simulink model "Both_Test_v3"  (R2017b)
settings: Solver=VariableStepAuto  StartTime=0.0  StopTime=2  MaxStep=1e-4  RelTol=1e-3
undefined symbols (not defined in the file): sigbuilder_block
libraries: powerlib x18, nesl_utility x2, fl_lib x2, simulink x1
settings Model: Creator=paul.rogers  LastModifiedBy=acer8_000
settings OptimizationCC: BlockReduction=off  ConditionallyExecuteInputs=off  DefaultParameterBehavior=Inlined
settings DebuggingCC: AlgebraicLoopMsg=error  SingleTaskRateTransMsg=error
settings HardwareCC: ProdBitPerPointer=32  ProdBitPerSizeT=32  ProdBitPerPtrDiffT=32  ProdLargestAtomicFloat=None  ProdIntDivRoundTo=Undefined  ProdEndianess=Unspecified  ProdWordSize=32  ProdHWDeviceType=ASIC/FPGA->ASIC/FPGA  ProdEqTarget=off
settings CodeAppCC: StateflowObjectComments=on
settings SimscapeCC: SimscapeNormalizeSystem=off

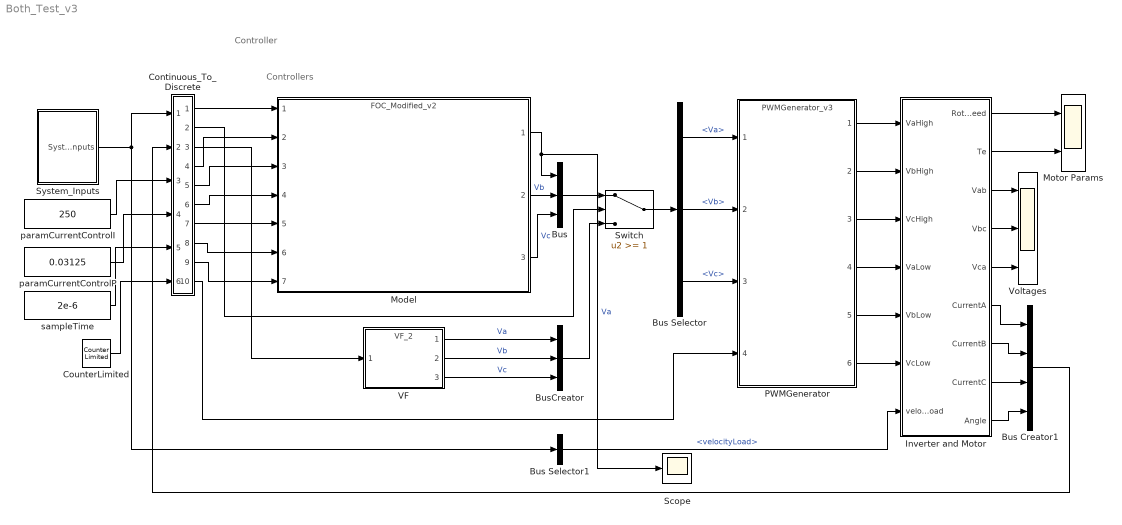
== system Both_Test_v3 ==
  note: Controllers
  note: Controller
  Bus : BusCreator  Inputs=3
  Bus Creator1 : BusCreator  Inputs=4
  Bus Selector : BusSelector  OutputSignals=Va,Vb,Vc
  Bus Selector1 : BusSelector  OutputSignals=velocityLoad
  BusCreator : BusCreator  Inputs=3
  Continuous_To_Discrete : Subsystem
      mask Display: fprintf('C/D')
  CounterLimited : simulink/Sources/Counter Limited  uplimit=50  tsamp=1e-5
  Inverter and Motor : Subsystem
  Model : ModelReference  ModelNameDialog=FOC_Modified_v2.slx  SimulationMode=Normal  ModelReferenceVersion=1.83
  Motor Params : Scope  NumInputPorts=2
  PWMGenerator : ModelReference  ModelNameDialog=PWMGenerator_v3.slx  SimulationMode=Normal  ModelReferenceVersion=1.20
  Scope : Scope
  Switch : Switch  Threshold=1
  System_Inputs : Subsystem  Description=""
      mask Display: disp('System\nInputs')
  VF : ModelReference  ModelNameDialog=VF_2.slx  SimulationMode=Normal  ModelReferenceVersion=1.58
  "Voltages " : Scope  NumInputPorts=3
  paramCurrentControlI : Constant  Value=250  OutDataTypeStr=fixdt(1,16,3)
  paramCurrentControlP : Constant  Value=0.03125  OutDataTypeStr=fixdt(1,16,8)
  sampleTime : Constant  Value=2e-6  OutDataTypeStr=fixdt(1,16,30)
  wires:
  Inverter and Motor/9(Angle) -> Bus Creator1/4
  Inverter and Motor/8(CurrentC) -> Bus Creator1/3
  Inverter and Motor/6(CurrentA) -> Bus Creator1/1
  Inverter and Motor/7(CurrentB) -> Bus Creator1/2
  paramCurrentControlP/1 -> Continuous_To_Discrete/4(paramCurrentControlP)
  paramCurrentControlI/1 -> Continuous_To_Discrete/3(paramCurrentControlI)
  System_Inputs/1(System_Inputs) -> Continuous_To_Discrete/1(System_Inputs), Bus Selector1/1
  Bus Creator1/1 -> Continuous_To_Discrete/2(Motor_Measurements)
  sampleTime/1 -> Continuous_To_Discrete/5(sampleTime)
  Bus Selector1/1 -> Inverter and Motor/7(velocityLoad)  "<velocityLoad>"
  Inverter and Motor/2(Te) -> Motor Params/2
  Inverter and Motor/1(Rotor Speed) -> Motor Params/1
  Inverter and Motor/3(Vab) -> "Voltages "/1
  Inverter and Motor/4(Vbc) -> "Voltages "/2
  Inverter and Motor/5(Vca) -> "Voltages "/3
  PWMGenerator/1 -> Inverter and Motor/1(VaHigh)
  PWMGenerator/2 -> Inverter and Motor/2(VbHigh)
  PWMGenerator/3 -> Inverter and Motor/3(VcHigh)
  PWMGenerator/4 -> Inverter and Motor/4(VaLow)
  PWMGenerator/5 -> Inverter and Motor/5(VbLow)
  PWMGenerator/6 -> Inverter and Motor/6(VcLow)
  CounterLimited/1 -> Continuous_To_Discrete/6(Counter)
  Continuous_To_Discrete/10(Counter_timed) -> PWMGenerator/4
  Switch/1 -> Bus Selector/1
  Bus Selector/3 -> PWMGenerator/3  "<Vc>"
  Bus Selector/1 -> PWMGenerator/1  "<Va>"
  Bus Selector/2 -> PWMGenerator/2  "<Vb>"
  Bus/1 -> Switch/1
  Model/1 -> Scope/1, Bus/1  "Va"
  Model/2 -> Bus/2  "Vb"
  Model/3 -> Bus/3  "Vc"
  Continuous_To_Discrete/9(sampleTime_timed) -> Model/7
  Continuous_To_Discrete/8(paramCurrentControlP_timed) -> Model/6
  Continuous_To_Discrete/7(paramCurrentControlI_timed) -> Model/5
  Continuous_To_Discrete/6(Electrical_Position) -> Model/4
  Continuous_To_Discrete/5(Phase_Current_B) -> Model/3
  Continuous_To_Discrete/4(Phase_Current_A) -> Model/2
  Continuous_To_Discrete/1(Current_Command) -> Model/1
  Continuous_To_Discrete/3(Frequency) -> VF/1
  Continuous_To_Discrete/2(Switch) -> Switch/2
  VF/3 -> BusCreator/3  "Vc"
  VF/2 -> BusCreator/2  "Vb"
  BusCreator/1 -> Switch/3
  VF/1 -> BusCreator/1  "Va"

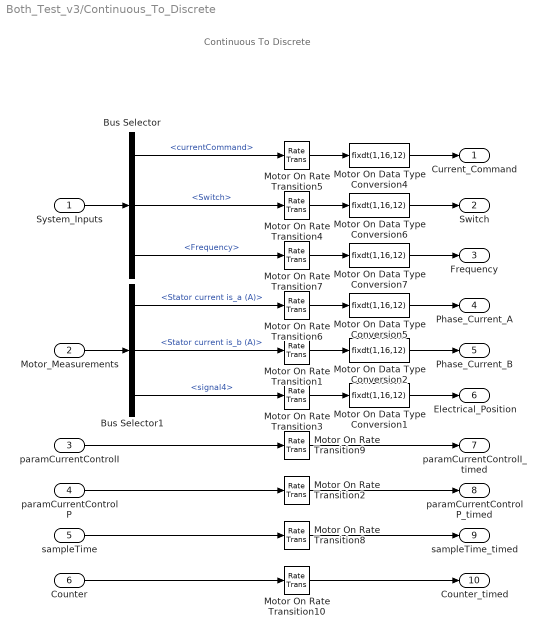
== system Both_Test_v3/Continuous_To_Discrete ==
  note: Continuous To Discrete
  System_Inputs : Inport
  Motor_Measurements : Inport  Port=2
  paramCurrentControlI : Inport  Port=3
  paramCurrentControlP : Inport  Port=4
  sampleTime : Inport  Port=5
  Counter : Inport  Port=6  OutDataTypeStr=uint8
  Bus Selector : BusSelector  OutputSignals=currentCommand,Switch,Frequency
  Bus Selector1 : BusSelector  OutputSignals=Stator current is_a (A),Stator current is_b (A),signal4
  Motor On Data Type Conversion{1..2,4..7} (6 alike) : DataTypeConversion  OutDataTypeStr=fixdt(1,16,12)
  Motor On Rate Transition{1..10} (10 alike) : RateTransition  Integrity=off  Deterministic=off  OutPortSampleTime=2e-6
  Current_Command : Outport
  Switch : Outport  Port=2
  Frequency : Outport  Port=3
  Phase_Current_A : Outport  Port=4
  Phase_Current_B : Outport  Port=5
  Electrical_Position : Outport  Port=6
  paramCurrentControlI_timed : Outport  Port=7
  paramCurrentControlP_timed : Outport  Port=8
  sampleTime_timed : Outport  Port=9
  Counter_timed : Outport  Port=10
  wires:
  Bus Selector1/3 -> Motor On Rate Transition3/1  "<signal4>"
  Bus Selector1/2 -> Motor On Rate Transition1/1  "<Stator current is_b (A)>"
  Bus Selector1/1 -> Motor On Rate Transition6/1  "<Stator current is_a (A)>"
  Motor On Data Type Conversion4/1 -> Current_Command/1
  Motor On Rate Transition6/1 -> Motor On Data Type Conversion5/1
  Motor On Rate Transition5/1 -> Motor On Data Type Conversion4/1
  Bus Selector/1 -> Motor On Rate Transition5/1  "<currentCommand>"
  Motor On Rate Transition3/1 -> Motor On Data Type Conversion1/1
  System_Inputs/1 -> Bus Selector/1
  Motor_Measurements/1 -> Bus Selector1/1
  Motor On Rate Transition1/1 -> Motor On Data Type Conversion2/1
  Motor On Rate Transition4/1 -> Motor On Data Type Conversion6/1
  Bus Selector/2 -> Motor On Rate Transition4/1  "<Switch>"
  Motor On Rate Transition7/1 -> Motor On Data Type Conversion7/1
  Bus Selector/3 -> Motor On Rate Transition7/1  "<Frequency>"
  Motor On Data Type Conversion6/1 -> Switch/1
  Motor On Data Type Conversion7/1 -> Frequency/1
  Motor On Data Type Conversion1/1 -> Electrical_Position/1
  Motor On Data Type Conversion2/1 -> Phase_Current_B/1
  Motor On Data Type Conversion5/1 -> Phase_Current_A/1
  paramCurrentControlI/1 -> Motor On Rate Transition9/1
  paramCurrentControlP/1 -> Motor On Rate Transition2/1
  sampleTime/1 -> Motor On Rate Transition8/1
  Counter/1 -> Motor On Rate Transition10/1
  Motor On Rate Transition10/1 -> Counter_timed/1
  Motor On Rate Transition8/1 -> sampleTime_timed/1
  Motor On Rate Transition2/1 -> paramCurrentControlP_timed/1
  Motor On Rate Transition9/1 -> paramCurrentControlI_timed/1

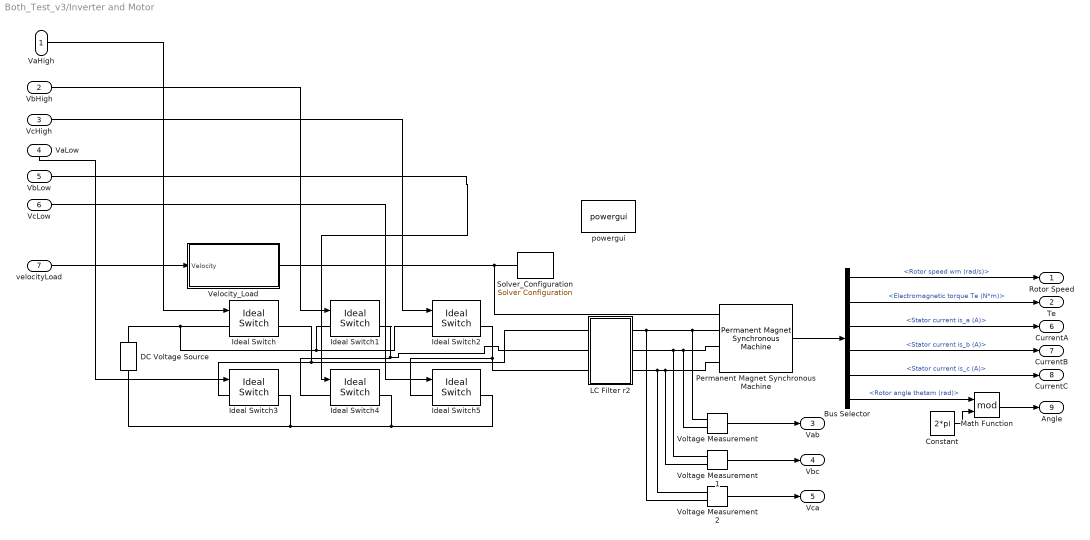
== system Both_Test_v3/Inverter and Motor ==
  VaHigh : Inport
  VbHigh : Inport  Port=2
  VcHigh : Inport  Port=3
  VaLow : Inport  Port=4
  VbLow : Inport  Port=5
  VcLow : Inport  Port=6
  velocityLoad : Inport  Port=7
  Bus Selector : BusSelector  OutputSignals=Rotor speed wm (rad/s),Electromagnetic torque Te (N*m),Stator current is_a (A),Stator current is_b (A),Stator current is_c (A),Rotor angle thetam (rad)
  Constant : Constant  Value=2*pi
  DC Voltage Source : powerlib/Electrical Sources/DC Voltage Source  Amplitude=42  Measurements=None
  Ideal Switch{,1..5} (6 alike) : powerlib/Power Electronics/Ideal Switch  Ron=0.001  Lon=0  IC=0  Rs=1e5  Cs=inf  Measurements=on
  LC Filter r2 : Subsystem  mask{L=10e-3, C=20e-6}
      mask prompts: L "Inductance"; C "Capacitance"
  Math Function : Math  Operator=mod  SaturateOnIntegerOverflow=on
  Permanent Magnet Synchronous Machine : powerlib/Machines/Permanent Magnet Synchronous Machine  NbPhases=3  FluxDistribution=Sinusoidal  RotorType=Salient-pole  MechanicalLoad=Mechanical rotational port  PresetModel=No  ShowDetailedParameters=on  MeasurementBus=off  Resistance=0.900000000000000  Inductance=8.5e-3  dqInductances=[0.001050000000000 0.001050000000000]  La=0.00049  MachineConstant=Torque Constant (N.m / A_peak)  Flux=0.005661  VoltageCst=4.1072  TorqueCst=0.033966007400000  Flat=120  Mechanical=[2.400927680000000e-06, 1.333630000000000e-05, 4, 0.002130661000000]  PolePairs=4  InitialConditions=[0,0, 0,0]  InitialConditions5ph=[0 0 0 0 0 0]  TsPowergui=0  TsBlock=-1  RefAngle=Aligned with phase A axis (original Park)
      settings: SourceProductName=Simscape Power Systems
  Solver_Configuration : nesl_utility/Solver Configuration  PhysicalDomain=network_engine_domain  SubClassName=solver  LeftPortType=input  RightPortType=generic  Accelerate=off  Tones=[]  Harmonics=[]  SimulateNoise=off  Profile=off  UseLocalSampling=off  EnableSwitchedLinearOptims=on  FrequencyDomain=off  UseCCode=off  RelTol=0.001  AbsTol=1e-06  MinStep=1e-09  ToWorkspace=off  RevertToSquareIcSolve=off  NumHomotopyIterations=100  PhasorMode=off  PhasorModeNumHarmonics=1  DoDC=off  ResidualTolerance=1e-9  UseLocalSolver=off  LocalSolverChoice=NE_BACKWARD_EULER_ADVANCER  LocalSolverSampleTime=.001  DoFixedCost=off  MaxNonlinIter=3  MaxModeIter=2  LinearAlgebra=Sparse  DelaysMemoryBudget=1024  AutomaticFiltering=on  FilteringTimeConstant=0.001
  Velocity_Load : Subsystem  VariantControl=loadType == motorLoad.disc
      mask Display:
      | image('hdlcoderVelocityLoadMask.png')
      | text(0.03, 0.5, '\omega', 'HorizontalAlignment', 'Left', 'texmode','on')
      | text(0.98, 0.5, 'R', 'HorizontalAlignment', 'Right')
  Voltage Measurement : powerlib/Measurements/Voltage Measurement  PhasorSimulation=off  OutputType=Complex  PSBequivalent=0
  Voltage Measurement1 : powerlib/Measurements/Voltage Measurement  PhasorSimulation=off  OutputType=Complex  PSBequivalent=0
  Voltage Measurement2 : powerlib/Measurements/Voltage Measurement  PhasorSimulation=off  OutputType=Complex  PSBequivalent=0
  powergui : powerlib/powergui  Priority=1  SimulationMode=Continuous  SampleTime=50e-6  frequency=60  Iterations=50  frequencyindice=0  Pbase=100e6  ErrMax=1e-4  UnitsV=kV  UnitsW=MW  buscounter=0  FunctionMessages=off  echomessages=off  EnableUseOfTLC=off  CurrentSourceSwitches=off  DisableSnubberDevices=off  DisableRonSwitches=off  DisableVfSwitches=off  DisplayEquations=off  SolverType=Tustin/Backward Euler (TBE)  Interpol=off  ExternalGateDelay=off  methode=off  Ts=100  x0status=blocks  SPID=on  SwTol=0  HookPort=off  RestoreLinks=warning  ResistiveCurrentMeasurement=off  Frange=[0:2:500]  Ylog=off  Xlog=on  ShowGrid=off  save=off  variable=ZData  structure=0  ZoomFFT=off  StartTime=0.0  cycles=1  DisplayStyle=1  fundamental=60  FreqAxis=off  MaxFrequency=1000  frequencyindicesteady=1  RmsSteady=1  display=off
  Rotor Speed : Outport
  Te : Outport  Port=2
  Vab : Outport  Port=3
  Vbc : Outport  Port=4
  Vca : Outport  Port=5
  CurrentA : Outport  Port=6
  CurrentB : Outport  Port=7
  CurrentC : Outport  Port=8
  Angle : Outport  Port=9
  wires:
  VbHigh/1 -> Ideal Switch1/1
  VcHigh/1 -> Ideal Switch2/1
  VcLow/1 -> Ideal Switch5/1
  VbLow/1 -> Ideal Switch4/1
  Permanent Magnet Synchronous Machine/1 -> Bus Selector/1
  Bus Selector/1 -> Rotor Speed/1  "<Rotor speed wm (rad/s)>"
  Bus Selector/2 -> Te/1  "<Electromagnetic torque Te (N*m)>"
  VaHigh/1 -> Ideal Switch/1
  Voltage Measurement2/1 -> Vca/1
  Voltage Measurement/1 -> Vab/1
  Voltage Measurement1/1 -> Vbc/1
  VaLow/1 -> Ideal Switch3/1
  Bus Selector/3 -> CurrentA/1  "<Stator current is_a (A)>"
  Bus Selector/4 -> CurrentB/1  "<Stator current is_b (A)>"
  Bus Selector/5 -> CurrentC/1  "<Stator current is_c (A)>"
  Bus Selector/6 -> Math Function/1  "<Rotor angle thetam (rad)>"
  Math Function/1 -> Angle/1
  Constant/1 -> Math Function/2
  velocityLoad/1 -> Velocity_Load/1(Velocity)
  connections:
  DC Voltage Source/RConn1 -- Ideal Switch2/LConn1 -- Ideal Switch1/LConn1 -- Ideal Switch/LConn1
  Ideal Switch2/RConn1 -- LC Filter r2/LConn3 -- Ideal Switch5/LConn1
  Ideal Switch1/RConn1 -- LC Filter r2/LConn2 -- Ideal Switch4/LConn1
  Ideal Switch/RConn1 -- LC Filter r2/LConn1 -- Ideal Switch3/LConn1
  DC Voltage Source/LConn1 -- Ideal Switch5/RConn1 -- Ideal Switch4/RConn1 -- Ideal Switch3/RConn1
  Solver_Configuration/RConn1 -- Permanent Magnet Synchronous Machine/LConn1 -- Velocity_Load/RConn1
  LC Filter r2/RConn1 -- Voltage Measurement2/LConn2 -- Voltage Measurement/LConn1 -- Permanent Magnet Synchronous Machine/LConn2
  LC Filter r2/RConn2 -- Voltage Measurement1/LConn1 -- Voltage Measurement/LConn2 -- Permanent Magnet Synchronous Machine/LConn3
  LC Filter r2/RConn3 -- Voltage Measurement2/LConn1 -- Voltage Measurement1/LConn2 -- Permanent Magnet Synchronous Machine/LConn4

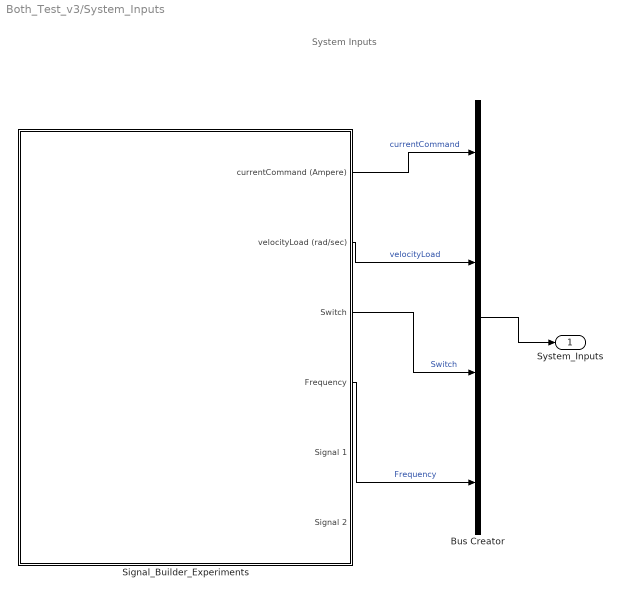
== system Both_Test_v3/System_Inputs ==
  note: System Inputs
  Bus Creator : BusCreator  Inputs=4
  Signal_Builder_Experiments : Subsystem  Tag=STV Subsys  LoadFcn=sigbuilder_block('load',[6 23.25 1428 723 ]);  StartFcn=sigbuilder_block('start');  StopFcn=sigbuilder_block('stop');  ClipboardFcn=sigbuilder_block('clipboard');  mask(Sigbuilder block){tuvar=[0:10]}
      mask init:
      | if ~strcmp(get_param(bdroot(gcb),'SimulationStatus'),'stopped'),tuvar = sigbuilder_block('maskInit'); end
      settings: CopyFcn=sigbuilder_block('copy');  DeleteFcn=sigbuilder_block('delete');  ModelCloseFcn=sigbuilder_block('modelClose');  PreSaveFcn=sigbuilder_block('preSave');  PauseFcn=sigbuilder_block('pause');  ContinueFcn=sigbuilder_block('continue');  NameChangeFcn=sigbuilder_block('namechange');  OpenFcn=sigbuilder_block('open',[6 23.25 1428 723 ]);  CloseFcn=sigbuilder_block('close');
      mask Display: plot(0, 0, 100, 100,[2, 2, 32, 32, 2], [68, 8, 8, 68, 68],[32, 2], [38, 38], [32, 19, 2],[53, 60, 44], [32, 17, 17, 2],[16, 16, 31, 31]);txt = getActiveGroup(gcbh);text(2, 100, txt,'verticalAlignment', 'top');
  System_Inputs : Outport
  wires:
  Signal_Builder_Experiments/2(velocityLoad (rad/sec)) -> Bus Creator/2  "velocityLoad"
  Signal_Builder_Experiments/1(currentCommand (Ampere)) -> Bus Creator/1  "currentCommand"
  Bus Creator/1 -> System_Inputs/1
  Signal_Builder_Experiments/3(Switch) -> Bus Creator/3  "Switch"
  Signal_Builder_Experiments/4(Frequency) -> Bus Creator/4  "Frequency"

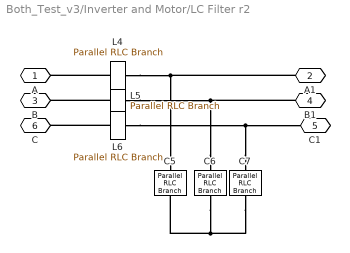
== system Both_Test_v3/Inverter and Motor/LC Filter r2 ==
  C5 : powerlib/Elements/Parallel RLC Branch  LConnTagsString=a  RConnTagsString=__new0  BranchType=C  Resistance=inf  Inductance=inf  SetiL0=off  InitialCurrent=0  Capacitance=C  Setx0=off  InitialVoltage=0  Measurements=None
  C6 : powerlib/Elements/Parallel RLC Branch  LConnTagsString=a  RConnTagsString=__new0  BranchType=C  Resistance=inf  Inductance=inf  SetiL0=off  InitialCurrent=0  Capacitance=C  Setx0=off  InitialVoltage=0  Measurements=None
  C7 : powerlib/Elements/Parallel RLC Branch  LConnTagsString=a  RConnTagsString=__new0  BranchType=C  Resistance=inf  Inductance=inf  SetiL0=off  InitialCurrent=0  Capacitance=C  Setx0=off  InitialVoltage=0  Measurements=None
  L4 : powerlib/Elements/Parallel RLC Branch  LConnTagsString=a  RConnTagsString=__new0  BranchType=L  Resistance=inf  Inductance=L  SetiL0=off  InitialCurrent=0  Capacitance=1.3e-3  Setx0=off  InitialVoltage=0  Measurements=None
  L5 : powerlib/Elements/Parallel RLC Branch  LConnTagsString=a  RConnTagsString=__new0  BranchType=L  Resistance=inf  Inductance=L  SetiL0=off  InitialCurrent=0  Capacitance=1.3e-3  Setx0=off  InitialVoltage=0  Measurements=None
  L6 : powerlib/Elements/Parallel RLC Branch  LConnTagsString=a  RConnTagsString=__new0  BranchType=L  Resistance=inf  Inductance=L  SetiL0=off  InitialCurrent=0  Capacitance=1.3e-3  Setx0=off  InitialVoltage=0  Measurements=None
  A : PMIOPort  Port=1  Side=Left
  A1 : PMIOPort  Port=2  Side=Right
  B : PMIOPort  Port=3  Side=Left
  B1 : PMIOPort  Port=4  Side=Right
  C1 : PMIOPort  Port=5  Side=Right
  C : PMIOPort  Port=6  Side=Left
  connections:
  L4/LConn1 -- A/RConn1
  L6/LConn1 -- C/RConn1
  C5/RConn1 -- C7/RConn1 -- C6/RConn1
  L5/LConn1 -- B/RConn1
  C6/LConn1 -- B1/RConn1 -- L5/RConn1
  L4/RConn1 -- A1/RConn1 -- C5/LConn1
  C7/LConn1 -- C1/RConn1 -- L6/RConn1

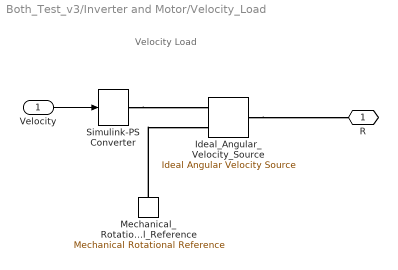
== system Both_Test_v3/Inverter and Motor/Velocity_Load ==
  note: Velocity Load
  Velocity : Inport
  Ideal_Angular_Velocity_Source : fl_lib/Mechanical/Mechanical Sources/Ideal Angular Velocity Source
  Mechanical_Rotational_Reference : fl_lib/Mechanical/Rotational Elements/Mechanical Rotational Reference
  Simulink-PS Converter : nesl_utility/Simulink-PS Converter  PhysicalDomain=network_engine_domain  SubClassName=ps_input  LeftPortType=input  RightPortType=output  PseudoPeriodic=off  Frequencies=[]  NoiseDistribution=none  NoiseParameters=[]  Unit=rad/s  AffineConversion=off  FilteringAndDerivatives=filter  SimscapeFilterOrder=1  InputFilterTimeConstant=.001  UdotUserProvided=1
  R : PMIOPort  Port=1  Side=Right
  wires:
  Velocity/1 -> Simulink-PS Converter/1
  connections:
  Ideal_Angular_Velocity_Source/LConn1 -- R/RConn1
  Simulink-PS Converter/RConn1 -- Ideal_Angular_Velocity_Source/RConn1
  Mechanical_Rotational_Reference/LConn1 -- Ideal_Angular_Velocity_Source/RConn2

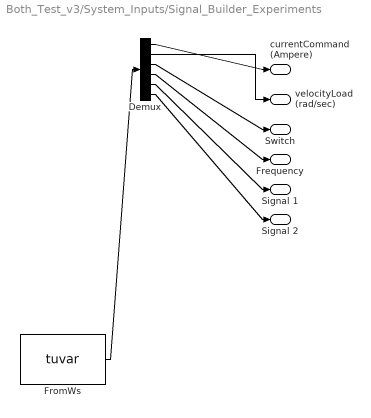
== system Both_Test_v3/System_Inputs/Signal_Builder_Experiments ==
  Demux : Demux  Tag=STV Demux  Outputs=6
  FromWs : FromWorkspace  Tag=STV FromWs  VariableName=tuvar  SampleTime=0
      SigBuilderData=|
      | dataSet(1).timeRange = [0 3]
      | dataSet(1).name = '1 Amp step, locked rotor'
      | dataSet(2).timeRange = [0 3]
      | dataSet(2).name = '+/-1 Amp step, locked rotor'
      | dataSet(3).timeRange = [0 2]
      | dataSet(3).name = '1 Amp, +/-100 rad/sec step'
      | sbobj.Name = 'Signal Builder'
      | sbobj.Groups(1).Name = '1 Amp step, locked rotor'
      | sbobj.Groups(1).Signals(1).Name = 'currentCommand (Ampere)'
      | sbobj.Groups(1).Signals(1).XData = [0 0.05 0.05 0.8 0.8 3]
      | sbobj.Groups(1).Signals(1).YData = [0 0 1 1 0 0]
      | sbobj.Groups(1).Signals(2).Name = 'velocityLoad (rad/sec)'
      | sbobj.Groups(1).Signals(2).XData = [0 3]
      | sbobj.Groups(1).Signals(2).YData = [0 0]
      | sbobj.Groups(1).Signals(3).Name = 'Switch'
      | sbobj.Groups(1).Signals(3).XData = [0 0.5 0.5 3]
      | sbobj.Groups(1).Signals(3).YData = [0 0 1 1]
      | sbobj.Groups(1).Signals(4).Name = 'Frequency'
      | sbobj.Groups(1).Signals(4).XData = [0 3]
      | sbobj.Groups(1).Signals(4).YData = [0 0]
      | sbobj.Groups(1).Signals(5).Name = 'Signal 1'
      | sbobj.Groups(1).Signals(5).XData = [0 1.5 1.5 3]
      | sbobj.Groups(1).Signals(5).YData = [0 0 1 1]
      | sbobj.Groups(1).Signals(6).Name = 'Signal 2'
      | sbobj.Groups(1).Signals(6).XData = [0 1 1 3]
      | sbobj.Groups(1).Signals(6).YData = [0 0 1 1]
      | sbobj.Groups(1).TimeRange = [0 3]
      | sbobj.Groups(2).Name = '+/-1 Amp step, locked rotor'
      | sbobj.Groups(2).Signals(1).Name = 'currentCommand (Ampere)'
      | sbobj.Groups(2).Signals(1).XData = [0 0.05 0.05 0.5 0.5 0.8 0.8 3]
      | sbobj.Groups(2).Signals(1).YData = [0 0 1 1 -1 -1 0 0]
      | sbobj.Groups(2).Signals(2).Name = 'velocityLoad (rad/sec)'
      | sbobj.Groups(2).Signals(2).XData = [0 1 3]
      | sbobj.Groups(2).Signals(2).YData = [0 0 0]
      | sbobj.Groups(2).Signals(3).Name = 'Switch'
      | sbobj.Groups(2).Signals(3).XData = [0 0.5 0.5 3]
      | sbobj.Groups(2).Signals(3).YData = [0 0 1 1]
      | sbobj.Groups(2).Signals(4).Name = 'Frequency'
      | sbobj.Groups(2).Signals(4).XData = [0 3]
      | sbobj.Groups(2).Signals(4).YData = [0 0]
      | sbobj.Groups(2).Signals(5).Name = 'Signal 1'
      | sbobj.Groups(2).Signals(5).XData = [0 1.5 1.5 3]
      | sbobj.Groups(2).Signals(5).YData = [0 0 1 1]
      | sbobj.Groups(2).Signals(6).Name = 'Signal 2'
      | sbobj.Groups(2).Signals(6).XData = [0 1 1 3]
      | sbobj.Groups(2).Signals(6).YData = [0 0 1 1]
      | sbobj.Groups(2).TimeRange = [0 3]
      | sbobj.Groups(3).Name = '1 Amp, +/-100 rad/sec step'
      | sbobj.Groups(3).Signals(1).Name = 'currentCommand (Ampere)'
      | sbobj.Groups(3).Signals(1).XData = [0 0.8 2]
      | sbobj.Groups(3).Signals(1).YData = [1 1 1]
      | sbobj.Groups(3).Signals(2).Name = 'velocityLoad (rad/sec)'
      | sbobj.Groups(3).Signals(2).XData = [0 2]
      | sbobj.Groups(3).Signals(2).YData = [500 500]
      | sbobj.Groups(3).Signals(3).Name = 'Switch'
      | sbobj.Groups(3).Signals(3).XData = [0 1 1 2]
      | sbobj.Groups(3).Signals(3).YData = [0 0 1 1]
      | sbobj.Groups(3).Signals(4).Name = 'Frequency'
      | sbobj.Groups(3).Signals(4).XData = [0 2]
      | sbobj.Groups(3).Signals(4).YData = [500 500]
      | sbobj.Groups(3).Signals(5).Name = 'Signal 1'
      | sbobj.Groups(3).Signals(5).XData = [0 1.5 1.5 2]
      | sbobj.Groups(3).Signals(5).YData = [0 0 1 1]
      | sbobj.Groups(3).Signals(6).Name = 'Signal 2'
      | sbobj.Groups(3).Signals(6).XData = [0 1.5 1.5 2]
      | sbobj.Groups(3).Signals(6).YData = [30 30 10 10]
      | sbobj.Groups(3).TimeRange = [0 2]
  currentCommand (Ampere) : Outport  Tag=STV Outport
  velocityLoad (rad/sec) : Outport  Tag=STV Outport  Port=2
  Switch : Outport  Tag=STV Outport  Port=3
  Frequency : Outport  Tag=STV Outport  Port=4
  Signal 1 : Outport  Tag=STV Outport  Port=5
  Signal 2 : Outport  Tag=STV Outport  Port=6
  wires:
  Demux/2 -> velocityLoad (rad/sec)/1
  Demux/1 -> currentCommand (Ampere)/1
  FromWs/1 -> Demux/1
  Demux/3 -> Switch/1
  Demux/4 -> Frequency/1
  Demux/5 -> Signal 1/1
  Demux/6 -> Signal 2/1
